simulink model "stateflow_actionOrder"  (R2015b)
settings: Solver=FixedStepDiscrete  StartTime=0.0  StopTime=10.0  RelTol=1e-3
settings Model: Creator=amyyang  LastModifiedBy=amyyang
settings OptimizationCC: DefaultParameterBehavior=Inlined  OptimizeModelRefInitCode=on  LifeSpan=1
settings RTWCC: SystemTargetFile=ert.tlc  GenCodeOnly=on  TemplateMakefile=ert_default_tmf  Description=Embedded Coder  GenerateReport=on  IncludeHyperlinkInReport=on  LaunchReport=on  GenerateTraceInfo=on  GenerateTraceReport=on  GenerateTraceReportSl=on  GenerateTraceReportSf=on  GenerateTraceReportEml=on
settings CodeAppCC: IgnoreCustomStorageClasses=off
settings ERTTargetCC: GenerateSampleERTMain=on  InlinedParameterPlacement=NonHierarchical  ERTCustomFileTemplate=example_file_process.tlc

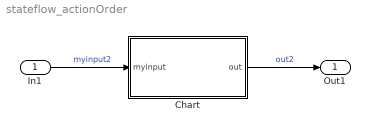
== system stateflow_actionOrder ==
  In1 : Inport
  Chart : Stateflow chart  TreatAsAtomicUnit=on
  Out1 : Outport
  wires:
  Chart/1(out) -> Out1/1  "out2"
  In1/1 -> Chart/1(myinput)  "myinput2"

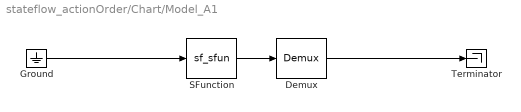
== system stateflow_actionOrder/Chart/Model_A1 ==
  " Demux " : Demux  Outputs=1
  " Ground " : Ground
  " SFunction " : S-Function  Tag=Stateflow S-Function stateflow_actionOrder 1  FunctionName=sf_sfun  PortCounts=[1 1]  SFunctionDeploymentMode=off  EnableBusSupport=off
  " Terminator " : Terminator
  wires:
  " Ground "/1 -> " SFunction "/1
  " Demux "/1 -> " Terminator "/1
  " SFunction "/1 -> " Demux "/1

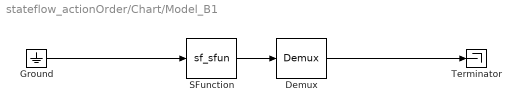
== system stateflow_actionOrder/Chart/Model_B1 ==
  " Demux " : Demux  Outputs=1
  " Ground " : Ground
  " SFunction " : S-Function  Tag=Stateflow S-Function stateflow_actionOrder 2  FunctionName=sf_sfun  PortCounts=[1 1]  SFunctionDeploymentMode=off  EnableBusSupport=off
  " Terminator " : Terminator
  wires:
  " Ground "/1 -> " SFunction "/1
  " Demux "/1 -> " Terminator "/1
  " SFunction "/1 -> " Demux "/1

== stateflow chart stateflow_actionOrder/Chart/Model_A1 ==
  state Off_A
  state On_A
  (default) -> Off_A
  Off_A -> On_A : [a]
  On_A -> Off_A : [~a]

== stateflow chart stateflow_actionOrder/Chart/Model_B1 ==
  state Off_A
  state On_A
  (default) -> Off_A
  Off_A -> On_A : [a]
  On_A -> Off_A : [~a]

== stateflow chart stateflow_actionOrder/Chart ==
  state Model_B
    state Off_B
    state On_B
    (default) -> Off_B
    Off_B -> On_B : [a]
    On_B -> Off_B : [~a]
  state Model_A
    state Off_A
    state On_A
    (default) -> Off_A
    Off_A -> On_A : [a]
    On_A -> Off_A : [~a]
  state Model_B1
  state Model_A1
  (default) -> Model_A [order 1]
  Model_A -> Model_B : [ condition]
  Model_B -> Model_A : [ condition]
  (default) -> Model_A1 [order 2]
  Model_A1 -> Model_B1 : [ condition]
  Model_B1 -> Model_A1 : [ condition]
  data: out output; myinput input; data local
